simulink model "total_sys"  (R2015a)
settings: Solver=ode45  StartTime=0.0  StopTime=20  RelTol=1e-3
values from neighbouring files (symbols this model uses):
  A = A    [design.m]    (also in init.mat = [2.98564337206 1 0 0 0 -3.00327796547 0 1 0 0 0.709627661926)
  B = B    [design.m]    (also in init.mat = [1 0 0 0 0])
  C = [-0.0746143795197 0.142131862116 0 0 0]    [init.mat]
  D = zeros(1+length(A(:,1)),1)    [design.m]    (also in init.mat = 0)
  H = [C;eye(size(A))]    [design.m]
  Ke = -3.8587    [init.mat]
  Kp = 35.7244    [init.mat]
undefined symbols (not defined in the file or in its folder): K, M, National_Instruments, PCI
libraries: sldrtlib x2
settings Model: Creator=João  LastModifiedBy=João

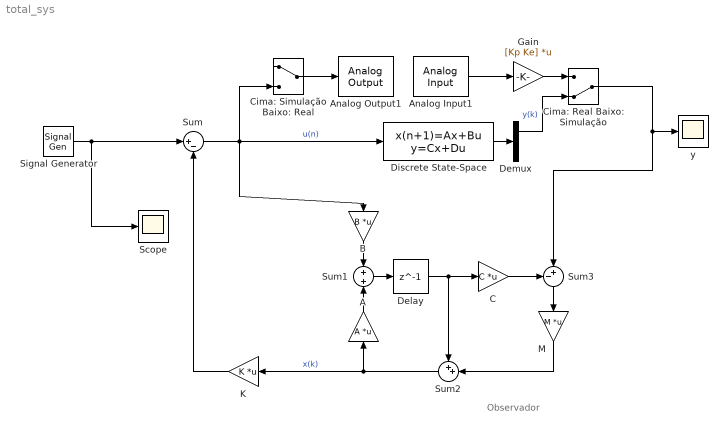
== system total_sys ==
  note: Observador
  A : Gain  Gain=A  Multiplication=Matrix(K*u) (u vector)
  Analog Input1 : sldrtlib/Analog Input  SampleTime=0.02  MaxMissedTicks=10  ShowMissedTicks=off  YieldWhenWaiting=off  DrvName=National_Instruments/PCI-6221  DrvAddress=4294967295  DrvOptions=[0 0 0 0 0]  Channels=[1 2]  RangeMode=1  VoltRange=1  DataType=1
      settings: AttributesFormatString=National Instruments\nPCI-6221 [auto]
  Analog Output1 : sldrtlib/Analog Output  SampleTime=0.02  MaxMissedTicks=10  ShowMissedTicks=off  YieldWhenWaiting=off  DrvName=National_Instruments/PCI-6221  DrvAddress=4294967295  DrvOptions=[0 0 0 0 0]  Channels=1  RangeMode=1  VoltRange=1  InitialValue=0  FinalValue=0
      settings: AttributesFormatString=National Instruments\nPCI-6221 [auto]
  B : Gain  Gain=B  Multiplication=Matrix(K*u) (u vector)
  C : Gain  Gain=C  Multiplication=Matrix(K*u) (u vector)
  Cima: Real Baixo: Simulação : ManualSwitch  CurrentSetting=0
  Cima: Simulação Baixo: Real : ManualSwitch
  Delay : Delay  DelayLength=1  InitialCondition=0  SampleTime=0.02
  Demux : Demux  Outputs=2
  Discrete State-Space : DiscreteStateSpace  A=A  B=B  C=H  D=D  SampleTime=0.02
  Gain : Gain  Gain=[Kp Ke]  Multiplication=Matrix(K*u) (u vector)
  K : Gain  Gain=K  Multiplication=Matrix(K*u) (u vector)
  M : Gain  Gain=M  Multiplication=Matrix(K*u) (u vector)
  Scope : Scope
      settings: SampleInput=on
  Signal Generator : SignalGenerator  Units=rad/sec
  Sum : Sum  Inputs=|+-
  Sum1 : Sum  Inputs=+|+
  Sum2 : Sum  Inputs=++|
  Sum3 : Sum  Inputs=-+|
  y : Scope
      settings: SampleInput=on
  wires:
  Sum/1 -> Discrete State-Space/1, B/1, Cima: Simulação Baixo: Real/2  "u(n)"
  B/1 -> Sum1/1
  Sum1/1 -> Delay/1
  A/1 -> Sum1/2
  Delay/1 -> C/1, Sum2/1
  C/1 -> Sum3/1
  Sum3/1 -> M/1
  M/1 -> Sum2/2
  Discrete State-Space/1 -> Demux/1
  Sum2/1 -> K/1, A/1  "x(k)"
  Signal Generator/1 -> Sum/1, Scope/1
  Gain/1 -> Cima: Real Baixo: Simulação/1
  Demux/1 -> Cima: Real Baixo: Simulação/2  "y(k)"
  Cima: Real Baixo: Simulação/1 -> Sum3/2, y/1
  Cima: Simulação Baixo: Real/1 -> Analog Output1/1
  Analog Input1/1 -> Gain/1
  K/1 -> Sum/2
